simulink model "rcam_simulation"  (R2022a)
settings: Solver=VariableStepAuto  StartTime=0.0  StopTime=60  RelTol=1e-3
values from neighbouring files (symbols this model uses):
  u1max = 25*pi/180    (= 0.436332312999)    [init.m]
  u1min = -25*pi/180    (= -0.436332312999)    [init.m]
  u2max = 10*pi/180    (= 0.174532925199)    [init.m]
  u2min = -25*pi/180    (= -0.436332312999)    [init.m]
  u3max = 30*pi/180    (= 0.523598775598)    [init.m]
  u3min = -30*pi/180    (= -0.523598775598)    [init.m]
  u4max = 10*pi/180    (= 0.174532925199)    [init.m]
  u5max = 10*pi/180    (= 0.174532925199)    [init.m]
  u5min = 0.5*pi/180    (= 0.00872664625997)    [init.m]
  x0 = [85 ... (first row only)    [init.m]
settings Model: Creator=dfl  LastModifiedBy=dfl

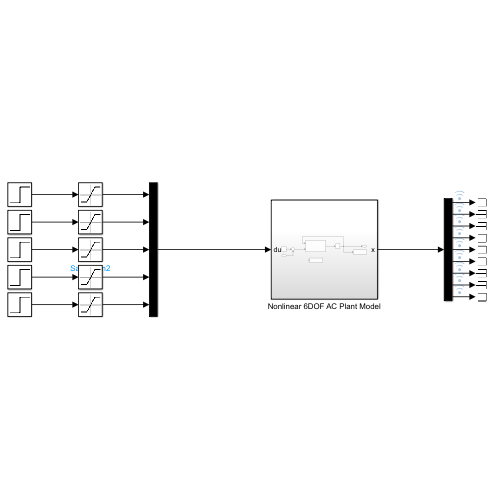
[thumbnail: Simulink's stored preview of the top-level diagram]
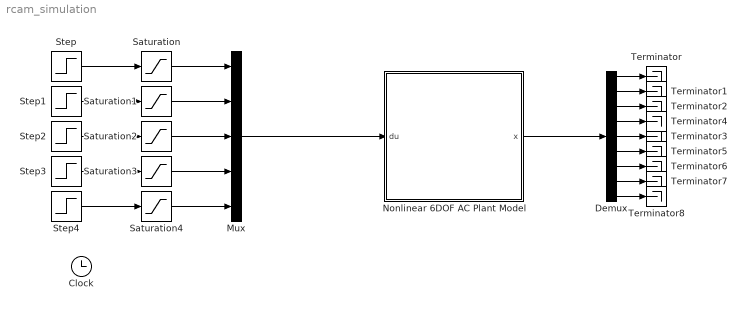
== system rcam_simulation ==
  Demux : Demux  Outputs=9
  Mux : Mux  Inputs=5
  Nonlinear 6DOF AC Plant Model : Subsystem
  Saturation : Saturate  UpperLimit=u1max  LowerLimit=u1min
  Saturation1 : Saturate  UpperLimit=u2max  LowerLimit=u2min
  Saturation2 : Saturate  UpperLimit=u3max  LowerLimit=u3min
  Saturation3 : Saturate  UpperLimit=u4max  LowerLimit=u3min
  Saturation4 : Saturate  UpperLimit=u5max  LowerLimit=u5min
  Step{,1..4} (5 alike) : Step  SampleTime=0
  Terminator{,1..8} (9 alike) : Terminator
  Clock : Clock
      settings: IOType=siggen
  wires:
  Nonlinear 6DOF AC Plant Model/1(x) -> Demux/1
  Step/1 -> Saturation/1
  Saturation/1 -> Mux/1
  Step1/1 -> Saturation1/1
  Saturation1/1 -> Mux/2
  Step2/1 -> Saturation2/1
  Saturation2/1 -> Mux/3
  Step3/1 -> Saturation3/1
  Saturation3/1 -> Mux/4
  Step4/1 -> Saturation4/1
  Saturation4/1 -> Mux/5
  Mux/1 -> Nonlinear 6DOF AC Plant Model/1(du)
  Demux/1 -> Terminator/1
  Demux/2 -> Terminator1/1
  Demux/3 -> Terminator2/1
  Demux/5 -> Terminator3/1
  Demux/4 -> Terminator4/1
  Demux/6 -> Terminator5/1
  Demux/7 -> Terminator6/1
  Demux/8 -> Terminator7/1
  Demux/9 -> Terminator8/1

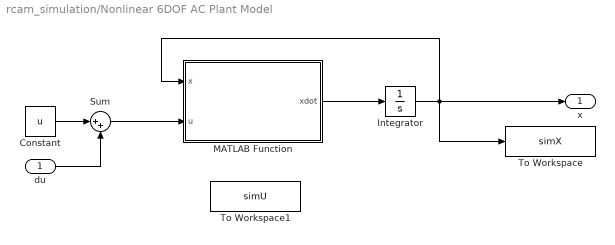
== system rcam_simulation/Nonlinear 6DOF AC Plant Model ==
  du : Inport
  Constant : Constant  Value=u
  Integrator : Integrator  InitialCondition=x0
  MATLAB Function : MATLAB Function  TreatAsAtomicUnit=on
  Sum : Sum  Inputs=|++
  To Workspace : ToWorkspace  VariableName=simX  SaveFormat=Timeseries  SampleTime=-1
  To Workspace1 : ToWorkspace  VariableName=simU  SaveFormat=Timeseries  SampleTime=-1
  x : Outport
  wires:
  Integrator/1 -> x/1, MATLAB Function/1(x), To Workspace/1
  MATLAB Function/1(xdot) -> Integrator/1
  Constant/1 -> Sum/1
  du/1 -> Sum/2
  Sum/1 -> MATLAB Function/2(u)

== matlab function rcam_simulation/Nonlinear 6DOF AC Plant Model/MATLAB Function ==
  data: x input; u input; xdot output
function xdot = plant_model(x, u)

xdot = rcam_model(x,u);
